simulink model "lab1"  (Simulink 7.9)
settings: Solver=ode45  StartTime=0.0  StopTime=10.0  RelTol=1e-3
settings Model: Creator=Mihail  LastModifiedBy=Mihail

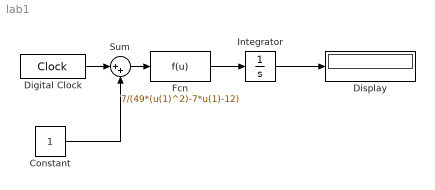
== system lab1 ==
  Constant : Constant
  Digital Clock : DigitalClock
  Display : Display
  Fcn : Fcn  Expr=7/(49*(u(1)^2)-7*u(1)-12)
  Integrator : Integrator
  Sum : Sum  Inputs=|++
  wires:
  Fcn/1 -> Integrator/1
  Integrator/1 -> Display/1
  Digital Clock/1 -> Sum/1
  Sum/1 -> Fcn/1
  Constant/1 -> Sum/2
